simulink model "v2_sim_PID"  (R2023b)
settings: Solver=VariableStepAuto  StartTime=0.0  StopTime=200  RelTol=1e-10
values from neighbouring files (symbols this model uses):
  C = 4.2975*(s+0.191)*(s+0.1311)/(s*(s+3.039))    [WP4.m]
libraries: simulink x2
settings Model: Creator=kiraa  LastModifiedBy=kiraa

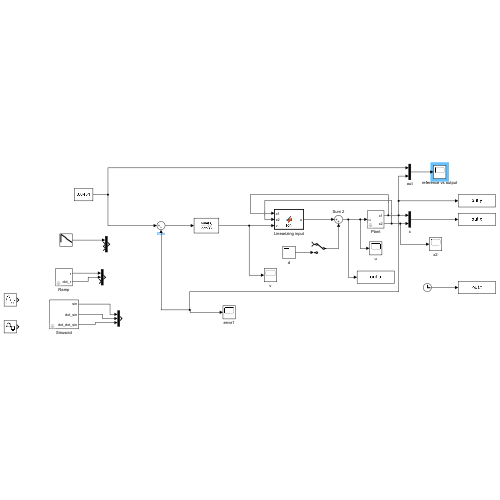
[thumbnail: Simulink's stored preview of the top-level diagram]
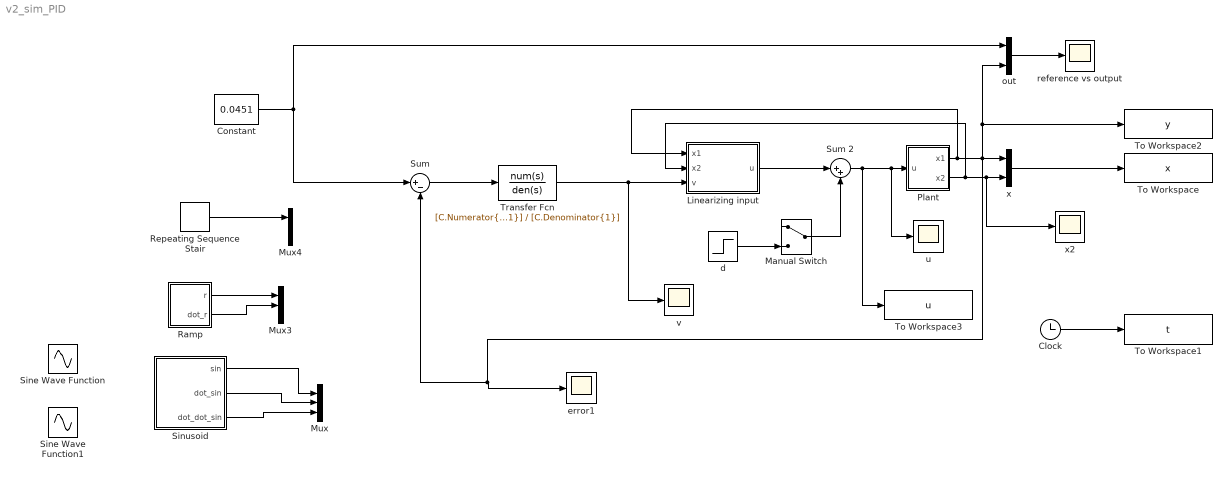
== system v2_sim_PID ==
  Clock : Clock
  Constant : Constant  Value=0.0451
  Linearizing input : MATLAB Function  TreatAsAtomicUnit=on
  Manual Switch : ManualSwitch
  Mux : Mux  Inputs=3
  Mux3 : Mux  Inputs=3
  Mux4 : Mux  Inputs=3
  Plant : Subsystem  mask{x1_0=0.1, x2_0=0}
      mask prompts: x1_0 "x1(0) [g/l]"; x2_0 "x2(0) [min^-1]"
  Ramp : Subsystem  mask{s=-0.0005, q=0.1}
      mask prompts: s "Slope"; q "Intercept"
  Repeating Sequence Stair : simulink/Sources/Repeating Sequence Stair  OutValues=[0.1:-0.01:0.01].'  tsamp=15  OutMin=[]  OutMax=[]  OutDataTypeStr=double  OutputDataTypeScalingMode=double  OutDataType=fixdt(0,8)  ConRadixGroup=Best Precision: Vector-wise  OutScaling=2^-12
  Sine Wave Function : Sin  Amplitude=0.005  Bias=0.0451  Frequency=0.3  SampleTime=0
  Sine Wave Function1 : Sin  Amplitude=0.001  Bias=0.0451  Frequency=0.1  Samples=1  SampleTime=2
  Sinusoid : Subsystem  mask{A=0.02, w=0.2, phi=pi/2, b=0.07}
      mask prompts: A "Amplitude"; w "Frequency [rad/s]"; phi "Phase"; b "Bias"
  Sum : Sum  Inputs=|+-
  Sum 2 : Sum  Inputs=|++
  To Workspace : ToWorkspace  VariableName=x  SampleTime=-1
  To Workspace1 : ToWorkspace  VariableName=t  SaveFormat=Timeseries  SampleTime=-1
  To Workspace2 : ToWorkspace  VariableName=y  SampleTime=-1
  To Workspace3 : ToWorkspace  VariableName=u  SampleTime=-1
  Transfer Fcn : TransferFcn  Numerator=[C.Numerator{1}]  Denominator=[C.Denominator{1}]
  d : Step  Time=30  After=-10  SampleTime=0
  error1 : Scope
  out : Mux  Inputs=2
  reference vs output : Scope
  u : Scope
  v : Scope
  x : Mux  Inputs=2
  x2 : Scope
  wires:
  Clock/1 -> To Workspace1/1
  x/1 -> To Workspace/1
  out/1 -> reference vs output/1
  Plant/2(x2) -> Linearizing input/2(x2), x2/1, x/2
  Sum 2/1 -> To Workspace3/1, Plant/1(u), u/1
  Manual Switch/1 -> Sum 2/2
  Linearizing input/1(u) -> Sum 2/1
  Sinusoid/1(sin) -> Mux/1
  Sinusoid/2(dot_sin) -> Mux/2
  Sinusoid/3(dot_dot_sin) -> Mux/3
  Ramp/1(r) -> Mux3/1
  Ramp/2(dot_r) -> Mux3/2
  Transfer Fcn/1 -> v/1, Linearizing input/3(v)
  Constant/1 -> out/1, Sum/1
  Repeating Sequence Stair/1 -> Mux4/1
  d/1 -> Manual Switch/2
  Sum/1 -> Transfer Fcn/1
  Plant/1(x1) -> Linearizing input/1(x1), Sum/2, error1/1, To Workspace2/1, out/2, x/1

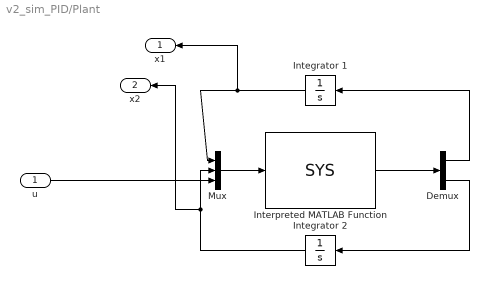
== system v2_sim_PID/Plant ==
  u : Inport
  Demux : Demux  Outputs=2
  Integrator 1 : Integrator  InitialCondition=x1_0
  Integrator 2 : Integrator  InitialCondition=x2_0
  Interpreted MATLAB Function : MATLABFcn  MATLABFcn=SYS  OutputDimensions=2
  Mux : Mux  Inputs=3
  x1 : Outport
  x2 : Outport  Port=2
  wires:
  Demux/1 -> Integrator 1/1
  Mux/1 -> Interpreted MATLAB Function/1
  Integrator 2/1 -> x2/1, Mux/2
  Interpreted MATLAB Function/1 -> Demux/1
  Demux/2 -> Integrator 2/1
  u/1 -> Mux/3
  Integrator 1/1 -> Mux/1, x1/1

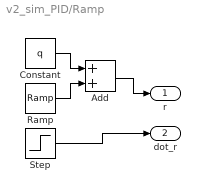
== system v2_sim_PID/Ramp ==
  Add : Sum
  Constant : Constant  Value=q
  Ramp : simulink/Sources/Ramp  slope=s  start=0  InitialOutput=0
  Step : Step  Time=0  After=s  SampleTime=0
  r : Outport
  dot_r : Outport  Port=2
  wires:
  Step/1 -> dot_r/1
  Ramp/1 -> Add/2
  Add/1 -> r/1
  Constant/1 -> Add/1

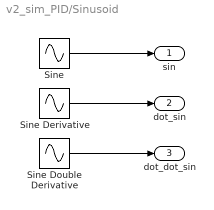
== system v2_sim_PID/Sinusoid ==
  Sine : Sin  Amplitude=A  Bias=b  Frequency=w  Phase=phi  SampleTime=0
  Sine Derivative : Sin  Amplitude=-A*w  Frequency=w  Phase=phi-pi/2  SampleTime=0
  Sine Double Derivative : Sin  Amplitude=-A*w*w  Frequency=w  Phase=phi  SampleTime=0
  sin : Outport
  dot_sin : Outport  Port=2
  dot_dot_sin : Outport  Port=3
  wires:
  Sine Derivative/1 -> dot_sin/1
  Sine/1 -> sin/1
  Sine Double Derivative/1 -> dot_dot_sin/1

== matlab function v2_sim_PID/Linearizing input ==
  data: x1 input; x2 input; v input; u output
function u = fcn(x1,x2,v)
    p1 = 0.0151; %tasso base di rimozione del glucosio dal sangue
    p2 = 0.0313; %tasso rimozione del glucosio dovuto all'insulina
    p3 = 0.0097;
    ge = 0.97;
    ie = 0.003;
    if x1 < 0.0000000001 %Messaggio di errore se lo stato x1 si annulla
        warning('The state x1 is approaching zero. This could led the system to explode.')
    end
    
    u = (1/(p3*x1))*((p1+x2)^2*x1-(p1+x2)*p1*ge+p2*x1*x2+p3*ie*x1-v);
    %fprintf("%.2f\n",u);
end
